simulink model "Simulink_UI_Test"  (R2025b)
settings: Solver=FixedStepAuto  StartTime=0.0  StopTime=inf  RelTol=1e-3
settings Model: SimulationMode=external  Creator=kueh_js  LastModifiedBy=kueh_js
settings OptimizationCC: OptimizeBlockIOStorage=off  EnhancedBackFolding=on  PassReuseOutputArgsThreshold=0.0  ZeroExternalMemoryAtStartup=off  ZeroInternalMemoryAtStartup=off  OptimizeBlockOrder=speed  DifferentSizesBufferReuse=on
settings DebuggingCC: ParameterTunabilityLossMsg=error
settings HardwareCC: ProdBitPerLong=64.0  ProdHWDeviceType=Intel->x86-64 (Linux 64)
settings SFSimCC: MATLABDynamicMemAlloc=off  SimTargetLang=C++  SimDLTargetLibrary=mkl-dnn
settings RTWCC: GenCodeOnly=on  Toolchain=GNU gcc/g++ | gmake (64-bit Linux)  TargetLang=C++
settings CodeAppCC: ForceParamTrailComments=on  OperatorAnnotations=on  MATLABSourceComments=on
settings GRTTargetCC: TargetLangStandard=C++20 (ISO)  MatFileLogging=off  CodeInterfacePackaging=C++ class

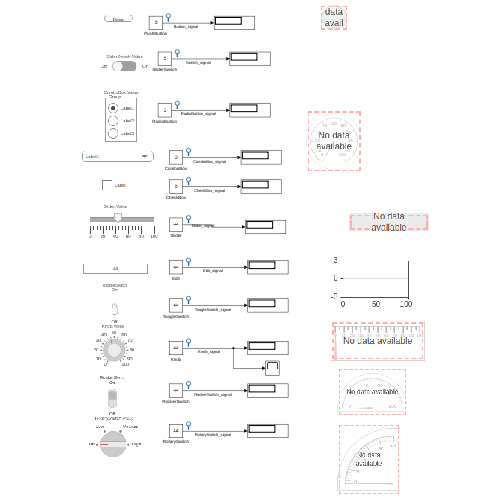
[thumbnail: Simulink's stored preview of the top-level diagram]
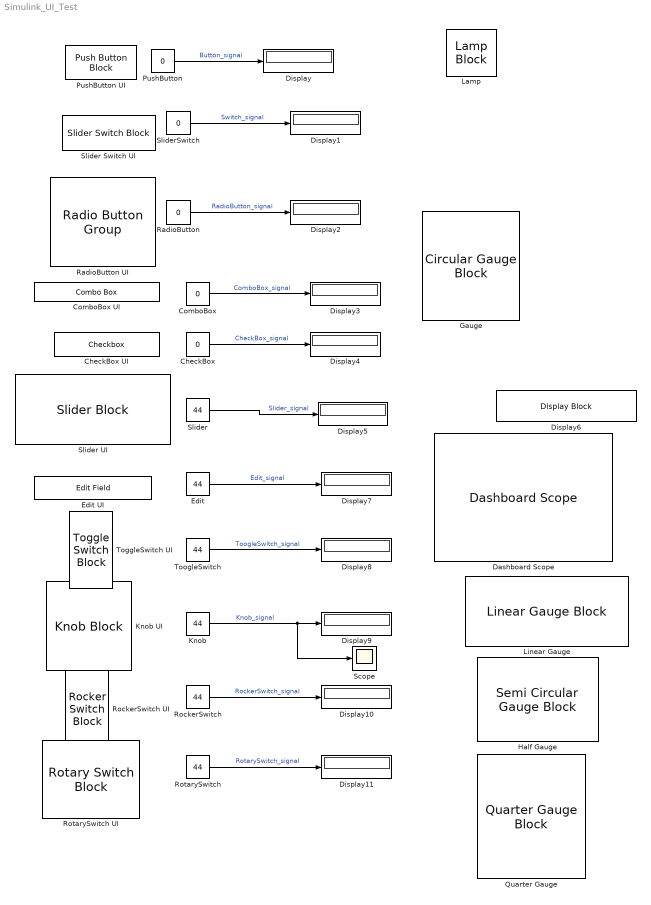
== system Simulink_UI_Test ==
  CheckBox : Constant  Value=0  OutDataTypeStr=boolean
  CheckBox UI : Checkbox  LabelPosition=Hide  ShowInitialText=on  Values=[0.0, 1.0]
  ComboBox : Constant  Value=0  OutDataTypeStr=boolean
  ComboBox UI : ComboBox  LabelPosition=Hide
  Dashboard Scope : DashboardScope  FontColor=[0.0, 0.0, 0.0]
  Display{,1..5,7..11} (11 alike) : Display
  Display6 : DisplayBlock  LabelPosition=Hide  Transparency=1  GridColor=[0.502, 0.502, 0.502]
  Edit : Constant  Value=44  OutDataTypeStr=boolean
  Edit UI : EditField  LabelPosition=Hide  ShowInitialText=on  Alignment=Center
  Gauge : CircularGaugeBlock  FontColor=[0.0, 0.0, 0.0]
  Half Gauge : SemiCircularGaugeBlock  FontColor=[0.0, 0.0, 0.0]
  Knob : Constant  Value=44  OutDataTypeStr=boolean
  Knob UI : KnobBlock
  Lamp : LampBlock  LabelPosition=Hide  DefaultColor=[192.0, 192.0, 192.0]
  Linear Gauge : LinearGaugeBlock  FontColor=[0.0, 0.0, 0.0]
  PushButton : Constant  Value=0  OutDataTypeStr=boolean
  PushButton UI : PushButtonBlock  ButtonText=Reset  IconOnColor=[0.0, 0.39215686274509803, 0.0]  IconOffColor=[0.0, 1.0, 0.0]  OffValue=0.000000
  Quarter Gauge : QuarterGaugeBlock  FontColor=[0.0, 0.0, 0.0]
  RadioButton : Constant  Value=0  OutDataTypeStr=boolean
  RadioButton UI : RadioButtonGroup  ButtonGroupName=Group
  RockerSwitch : Constant  Value=44  OutDataTypeStr=boolean
  RockerSwitch UI : RockerSwitchBlock
  RotarySwitch : Constant  Value=44  OutDataTypeStr=boolean
  RotarySwitch UI : RotarySwitchBlock
  Scope : Scope
  Slider : Constant  Value=44  OutDataTypeStr=boolean
  Slider Switch UI : SliderSwitchBlock
  Slider UI : SliderBlock
  SliderSwitch : Constant  Value=0  OutDataTypeStr=boolean
  ToggleSwitch UI : ToggleSwitchBlock
  ToogleSwitch : Constant  Value=44  OutDataTypeStr=boolean
  wires:
  Slider/1 -> Display5/1  "Slider_signal"
  ComboBox/1 -> Display3/1  "ComboBox_signal"
  CheckBox/1 -> Display4/1  "CheckBox_signal"
  PushButton/1 -> Display/1  "Button_signal"
  RadioButton/1 -> Display2/1  "RadioButton_signal"
  SliderSwitch/1 -> Display1/1  "Switch_signal"
  Edit/1 -> Display7/1  "Edit_signal"
  ToogleSwitch/1 -> Display8/1  "ToogleSwitch_signal"
  Knob/1 -> Scope/1, Display9/1  "Knob_signal"
  RockerSwitch/1 -> Display10/1  "RockerSwitch_signal"
  RotarySwitch/1 -> Display11/1  "RotarySwitch_signal"
